simulink model "MHH_BUOI2_bai1"  (R2020b)
settings: Solver=VariableStepAuto  StartTime=0.0  StopTime=10.0  MaxStep=0.01  RelTol=1e-3
values from neighbouring files (symbols this model uses):
  b = 0.2    [bai4.mat]
  k = 10    [bai4.mat]
  M = 1    [bai4.mat]
libraries: dspsrcs4 x1
settings Model: Creator=John Andrew  LastModifiedBy=John Andrew

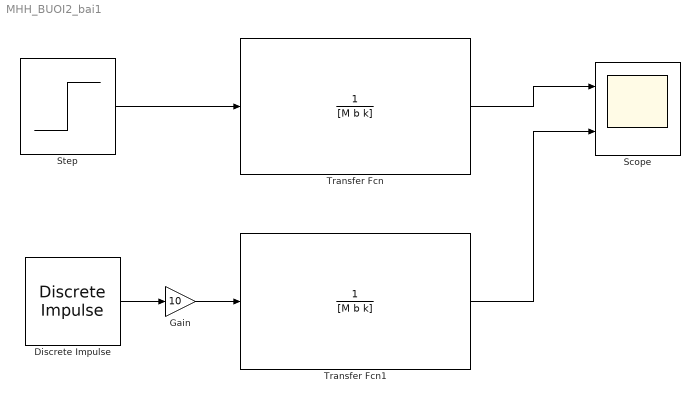
== system MHH_BUOI2_bai1 ==
  Discrete Impulse : dspsrcs4/Discrete  Impulse  Delay=1  SampleTime=1  FrameSample=1  OutputFrames=off  dataType=double  isSigned=on  wordLen=16  udDataType=sfix(16)  fracBitsMode=Best precision  numFracBits=15  OutDataTypeStr=double  LastOutDataTypeStr=double
  Gain : Gain  Gain=10
  Scope : Scope  NumInputPorts=2
  Step : Step  SampleTime=0
  Transfer Fcn : TransferFcn  Denominator=[M b k]
  Transfer Fcn1 : TransferFcn  Denominator=[M b k]
  wires:
  Transfer Fcn/1 -> Scope/1
  Step/1 -> Transfer Fcn/1
  Transfer Fcn1/1 -> Scope/2
  Discrete Impulse/1 -> Gain/1
  Gain/1 -> Transfer Fcn1/1
